simulink model "statechart"  (R2016b)
settings: Solver=VariableStepAuto  StartTime=0.0  StopTime=10  MaxStep=0.05  RelTol=1e-3
libraries: simulink x1, vrlib x1
settings Model: Creator=larry  LastModifiedBy=larry

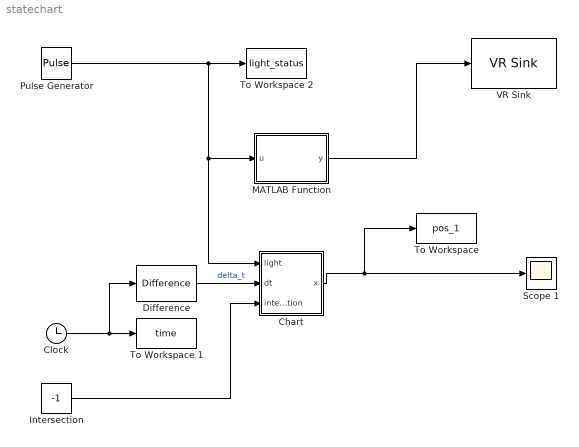
== system statechart ==
  Chart : Stateflow chart  TreatAsAtomicUnit=on
  Clock : Clock
  Difference : simulink/Discrete/Difference  ICPrevInput=0.0  OutMin=[]  OutMax=[]  OutDataType=fixdt(1, 16)  OutScaling=2^-10  DoSatur=off
  Intersection : Constant  Value=-1
  MATLAB Function : MATLAB Function  TreatAsAtomicUnit=on
  Pulse Generator : DiscretePulseGenerator  PulseType=Time based  Period=5  PulseWidth=50  PhaseDelay=1.5
  Scope 1 : Scope
  To Workspace : ToWorkspace  VariableName=pos_1  SampleTime=-1
  To Workspace 1 : ToWorkspace  VariableName=time  SampleTime=-1
  To Workspace 2 : ToWorkspace  VariableName=light_status  SampleTime=-1
  VR Sink : vrlib/VR Sink  InstantiateOnLoad=on  SampleTime=0.1  ViewEnable=on  RemoteChange=off  RemoteView=off  FieldsWritten=B1_material.diffuseColor.3.1.1.double  WorldFileName=test.wrl  AutoView=off  VideoDimensions=[]  AllowVariableSize=off
  wires:
  Pulse Generator/1 -> Chart/1(light), MATLAB Function/1(u), To Workspace 2/1
  Clock/1 -> Difference/1, To Workspace 1/1
  MATLAB Function/1(y) -> VR Sink/1
  Chart/1(x) -> To Workspace/1, Scope 1/1
  Difference/1 -> Chart/2(dt)  "delta_t"
  Intersection/1 -> Chart/3(intersection)

== matlab function statechart/MATLAB Function ==
  data: u input; y output
function y = fcn(u)

if u == 1
    y = [1 0 0];
else
    y = [0 1 0];
end

== stateflow chart statechart/Chart ==
  state Init
    entry:
    id = 1;
  state SpeedUp
    during:
    carAccelerate();
  state Stop
  state SlowDown
    during:
    carAccelerate();
  state FixRate
    during:
    x = x + v * 0.1;
  (default) -> Init
  Init -> Stop
  Stop -> SpeedUp : [~closeIntersect() || ...
      | greenLight()]/{a = 0.4;}
  SlowDown -> SpeedUp [order 2] : [~closeIntersect() ||...
      | greenLight()]/{a = 0.4;}
  SpeedUp -> SlowDown [order 2] : [stopByRedLight()]...
      | /{a = -0.4;}
  SpeedUp -> FixRate [order 1] : [v >= 1]/{ v = 1;}
  SlowDown -> Stop [order 1] : [v <= 1e-3]/{v = 0;}
  FixRate -> SlowDown : [stopByRedLight()]...
      | /{a = -0.4;}
  data: ra function_output; res function_output; res function_output; res function_output; res function_output; x output =-7.5; a local; v local =0; light input; dt input; intersection input double; id local
  function ra = accToStop:
    | function ra = accToStop
    | 
    | ra = -0.4;
  function res = stoppable:
    | function res = stoppable
    | 
    | res = true;
  function res = closeIntersect:
    | function res = closeIntersect
    | 
    | coder.extrinsic('evalin');
    | 
    | diff = intersection - x;
    | % diff = evalin('base', 'env.getIntersectDistByID(1)');
    | if diff >= 0 && diff <= 2
    |     res = true;
    | else
    |     res = false;
    | end
  function carAccelerate:
    | function carAccelerate
    | 
    | x = x + v * dt + 0.5 * a * dt * dt;
    | v = v + a * dt;
  function res = stopByRedLight:
    | function res = stopByRedLight
    | 
    | if closeIntersect() && light == 1
    |     res = true;
    | else
    |     res = false;
    | end
  function res = greenLight:
    | function res = greenLight
    | 
    | if light == 0
    |     res = true;
    | else 
    |     res = false;
    | end
